simulink model "newsim15"  (R2016a)
settings: Solver=VariableStepAuto  StartTime=0.0  StopTime=50  RelTol=1e-3
values from neighbouring files (symbols this model uses):
  A = [0 1 0 0; -k1/J1 -c1/J1 k1/J1 0;0 0 0 1; k1/J2 0 (-k1-k2)/J2 -c2/J2;]    [Controllable.m]    (also in ControllableV1.m = [0 1 0 0; ControllableV2.m = [0 1 0 0)
  B = [0; 1/J1; 0; 0;]    [Controllable.m]    (also in ControllableV1.m; ControllableV2.m)
  C = [1 0 0 0; 0 0 1 0]    [Controllable.m]    (also in ControllableV1.m = eye(4); ControllableV2.m = eye(4))
  D = [0;0]    [Controllable.m]    (also in ControllableV1.m = [0;0;0;0;]; ControllableV2.m = [0;0;0;0;])
  k = [k1 k2 k3 k4]    [Controllable.m]    (also in ControllableV1.m = kc / T; ControllableV2.m = kc / T)
settings Model: Creator=ramik  LastModifiedBy=ramik

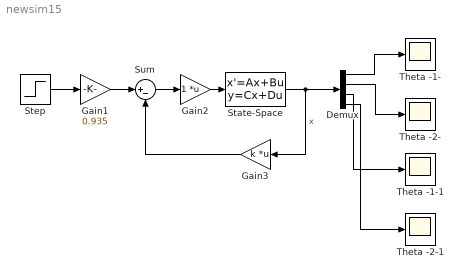
== system newsim15 ==
  Demux : Demux
  Gain1 : Gain  Gain=0.935  OutDataTypeStr=Inherit: Same as input
  Gain2 : Gain  Multiplication=Matrix(K*u)  OutDataTypeStr=Inherit: Same as input
  Gain3 : Gain  Gain=k  Multiplication=Matrix(K*u)  OutDataTypeStr=Inherit: Same as input
  State-Space : StateSpace  A=A  B=B  C=C  D=D  X0=0
  Step : Step  Time=0.001  After=1000  SampleTime=0.0001
  Sum : Sum  Inputs=|+-
  Theta -1- : Scope
  Theta -1-1 : Scope
  Theta -2- : Scope
  Theta -2-1 : Scope
  wires:
  Demux/1 -> Theta -1-/1
  Demux/2 -> Theta -2-/1
  State-Space/1 -> Gain3/1, Demux/1  "x"
  Step/1 -> Gain1/1
  Gain1/1 -> Sum/1
  Demux/4 -> Theta -2-1/1
  Demux/3 -> Theta -1-1/1
  Sum/1 -> Gain2/1
  Gain2/1 -> State-Space/1
  Gain3/1 -> Sum/2
